simulink model "mass_spring_damper"  (R2012b)
settings: Solver=ode4  StartTime=0.0  StopTime=10.0  FixedStep=sim_step  RelTol=1e-3
values from neighbouring files (symbols this model uses):
  h = 10    [msd_script.m]
  k = 10    [msd_script.m]
  m = 1    [msd_script.m]
  z = m*y(:,1)    [msd_script.m]
settings Model: Creator=c109799  LastModifiedBy=c109799

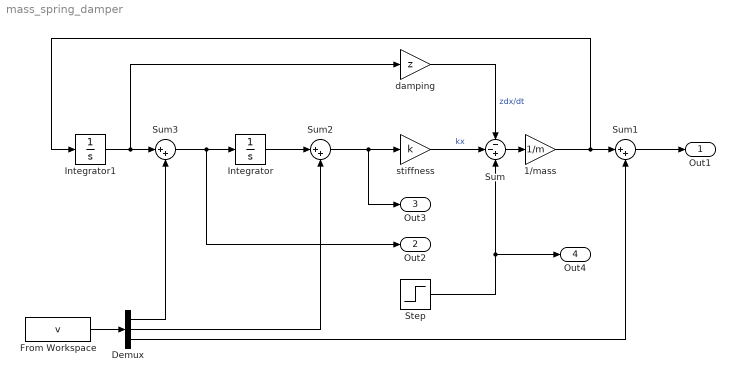
== system mass_spring_damper ==
  1/mass : Gain  Gain=1/m
  Demux : Demux  Outputs=3
  From Workspace : FromWorkspace  VariableName=v  SampleTime=0
  Integrator : Integrator  ContinuousStateAttributes='x'
  Integrator1 : Integrator  ContinuousStateAttributes='dx'
  Step : Step  After=h  SampleTime=0
  Sum : Sum  Inputs=--+
  Sum1 : Sum  Inputs=|++
  Sum2 : Sum  Inputs=|++
  Sum3 : Sum  Inputs=|++
  damping : Gain  Gain=z
  stiffness : Gain  Gain=k
  Out1 : Outport
  Out2 : Outport  Port=2
  Out3 : Outport  Port=3
  Out4 : Outport  Port=4
  wires:
  Integrator1/1 -> Sum3/1, damping/1
  stiffness/1 -> Sum/2  "kx"
  damping/1 -> Sum/1  "zdx/dt"
  Sum/1 -> 1/mass/1
  1/mass/1 -> Sum1/1, Integrator1/1
  Sum1/1 -> Out1/1
  Step/1 -> Out4/1, Sum/3
  Integrator/1 -> Sum2/1
  Sum3/1 -> Out2/1, Integrator/1
  From Workspace/1 -> Demux/1
  Demux/1 -> Sum3/2
  Demux/2 -> Sum2/2
  Demux/3 -> Sum1/2
  Sum2/1 -> Out3/1, stiffness/1
